simulink model "Benchmark2021ControllerNew"  (R2018a)
settings: Solver=ode1  StartTime=0  StopTime=t_end  FixedStep=simTs  RelTol=1e-3
values from neighbouring files (symbols this model uses):
  Horizon_Lowlayer = T_PreDomn-T_Apply    [Initial_Lower.m]
  Initial_headway = Sensor_FOL_dDist(2)    [Initial_main.m]
  Initial_MG1_spd = 0    [Initial_Lower.m]
  Initial_MG2_spd = 0    [Initial_Lower.m]
  Initial_SOC = 50    [Initial_main.m]
  Initial_vhcl_spd = 0    [Initial_main.m]
  N_opt = zeros(1,length(Power_ex))    [Initial_Lower.m]
  N_PMP_Lowlayer = Horizon_Lowlayer/Sampling_Lowlayer    [Initial_Lower.m]
  Power_level = 0:200:62800    [Initial_Lower.m]
  ras2rpm = 60/2/pi    (= 9.54929658551)    [Initial_main.m]
  Route_Destination_Distance = 16002    [Initial_Upper.m]
  rpm2rads = 1/rads2rpm    (= 0.10471975512)    [Initial_Lower.m]    (also in Initial_main.m)
  Sampling_Lowlayer = 0.05    [Initial_Lower.m]
  T_opt = zeros(1,length(Power_ex))    [Initial_Lower.m]
undefined symbols (not defined in the file or in its folder): DiscIntNeverNeededParam, Maxtorque_EngTrq, MG2_MaxMintorque_MaxTrq, MG2_MaxMintorque_Spd, Rc2, Rf1, Rf2, Rm, Rt, UpperLayerVpredict
(part 1 of 11)
settings Model: PauseTimes=100  Creator=1562880  LastModifiedBy=Lenovo
settings DataIOCC: SaveFormat=Structure  SaveOutput=off  SignalLogging=off  DSMLogging=off  SaveTime=off
settings OptimizationCC: BooleanDataType=off  DefaultParameterBehavior=Inlined  LifeSpan=1
settings DebuggingCC: SolverPrmCheckMsg=warning  FcnCallInpInsideContextMsg=warning  StateNameClashWarn=warning  SFUnexpectedBacktrackingDiag=warning  SFNoUnconditionalDefaultTransitionDiag=warning  SFExecutionAtInitializationDiag=none
settings CodeAppCC: StateflowObjectComments=on
settings GRTTargetCC: TargetLangStandard=C89/C90 (ANSI)  GeneratePreprocessorConditionals=Disable all
settings ConfigComp: CovMetricSettings=dw  CovHtmlReporting=on  CovSaveCumulativeToWorkspaceVar=on  CovSaveSingleToWorkspaceVar=on  CovExternalEMLEnable=off

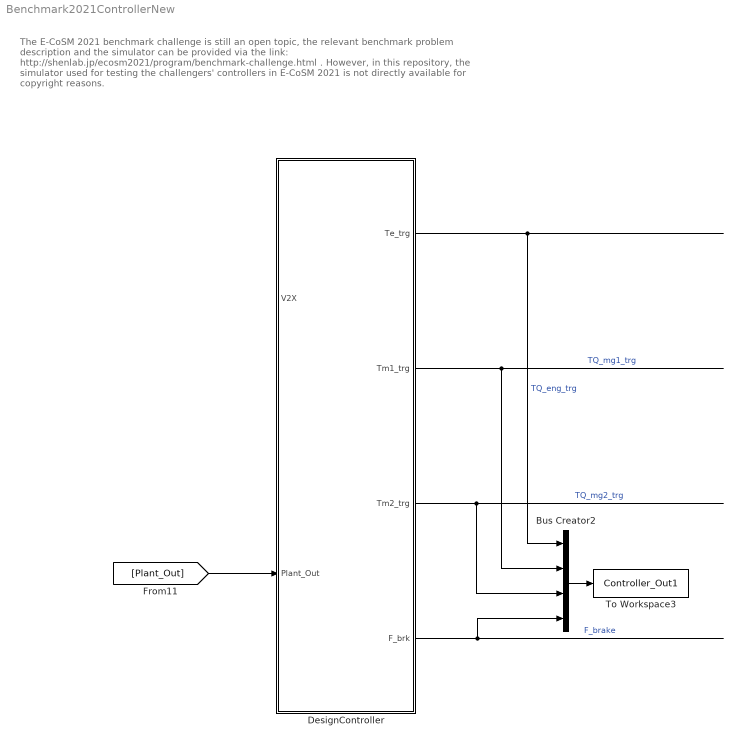
== system Benchmark2021ControllerNew ==
  note: The E-CoSM 2021 benchmark challenge is still an open topic, the relevant benchmark problem description and the simulator can be provided via the link: http://shenlab.jp/ecosm2021/program/benchmark-challenge.html . However, in this repository, the simulator used for testing the challengers' controllers in E-CoSM 2021 is not directly available for copyright reasons.
  Bus Creator2 : BusCreator  Inputs=4
  DesignController : Subsystem
  To Workspace3 : ToWorkspace  VariableName=Controller_Out1  SaveFormat=Timeseries  SampleTime=-1
  wires:
  [Plant_Out] -> DesignController/2(Plant_Out)
  DesignController/3(Tm2_trg) -> Bus Creator2/3  "TQ_mg2_trg"
  Bus Creator2/1 -> To Workspace3/1
  DesignController/1(Te_trg) -> Bus Creator2/1  "TQ_eng_trg"
  DesignController/4(F_brk) -> Bus Creator2/4  "F_brake"
  DesignController/2(Tm1_trg) -> Bus Creator2/2  "TQ_mg1_trg"

== system Benchmark2021ControllerNew/DesignController ==
  V2X : Inport
  Plant_Out : Inport  Port=2
  Benchmark-Controller : Subsystem
      mask Display: disp('JLU\nController')
  Te_trg : Outport
  Tm1_trg : Outport  Port=2
  Tm2_trg : Outport  Port=3
  F_brk : Outport  Port=4
  wires:
  V2X/1 -> Benchmark-Controller/1(V2X)  "Vel_trg"
  Benchmark-Controller/1(Te_trg) -> Te_trg/1
  Benchmark-Controller/2(Tm1_trg) -> Tm1_trg/1
  Benchmark-Controller/3(Tm2_trg) -> Tm2_trg/1
  Benchmark-Controller/4(F_brk) -> F_brk/1
  Plant_Out/1 -> Benchmark-Controller/2(Plant_Out)  "from E-CoSM plant-output"

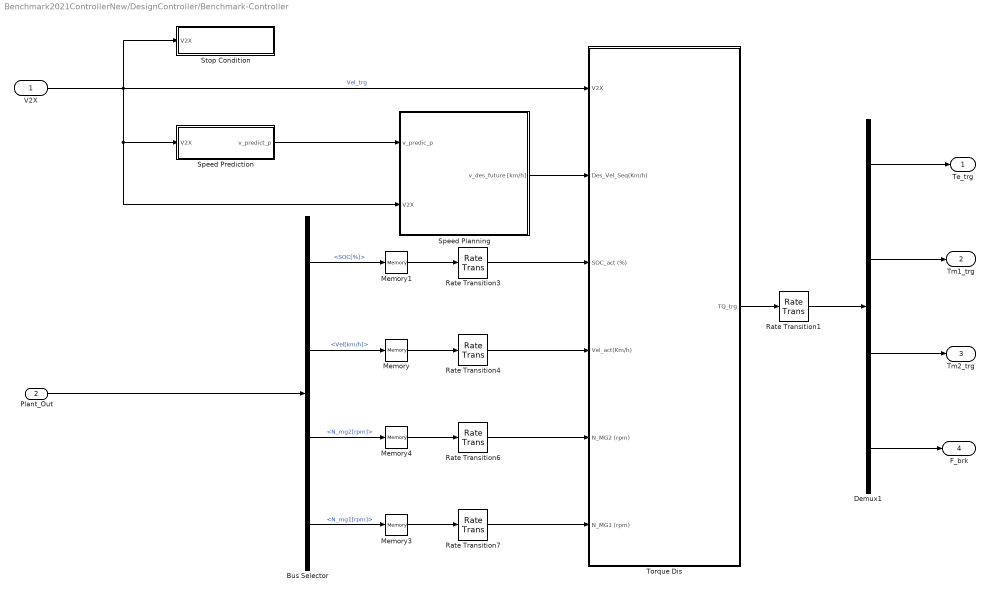
== system Benchmark2021ControllerNew/DesignController/Benchmark-Controller ==
  V2X : Inport
  Plant_Out : Inport  Port=2
  Bus Selector : BusSelector  OutputSignals=SOC[%],Vel[km/h],N_mg2[rpm],N_mg1[rpm]
  Demux1 : Demux
  Memory : Memory  InitialCondition=Initial_vhcl_spd
  Memory1 : Memory  InitialCondition=Initial_SOC
  Memory3 : Memory  InitialCondition=Initial_MG1_spd
  Memory4 : Memory  InitialCondition=Initial_MG2_spd
  Rate Transition1 : RateTransition  OutPortSampleTime=0.01
  Rate Transition3 : RateTransition  InitialCondition=50  OutPortSampleTime=0.05
  Rate Transition4 : RateTransition  OutPortSampleTime=0.05
  Rate Transition6 : RateTransition  OutPortSampleTime=0.05
  Rate Transition7 : RateTransition  OutPortSampleTime=0.05
  Speed Planning : Subsystem
  Speed Prediction : Subsystem  SystemSampleTime=0.05
  Stop Condition : Subsystem
  Torque Dis : Subsystem  SystemSampleTime=0.05
  Te_trg : Outport
  Tm1_trg : Outport  Port=2
  Tm2_trg : Outport  Port=3
  F_brk : Outport  Port=4
  wires:
  Speed Prediction/1(v_predict_p) -> Speed Planning/1(v_predic_p)
  V2X/1 -> Speed Planning/2(V2X), Speed Prediction/1(V2X), Stop Condition/1(V2X), Torque Dis/1(V2X)  "Vel_trg"
  Demux1/1 -> Te_trg/1
  Speed Planning/1(v_des_future [km/h]) -> Torque Dis/2(Des_Vel_Seq(Km/h))
  Torque Dis/1(TQ_trg) -> Rate Transition1/1
  Memory1/1 -> Rate Transition3/1
  Demux1/3 -> Tm2_trg/1
  Memory4/1 -> Rate Transition6/1
  Memory3/1 -> Rate Transition7/1
  Memory/1 -> Rate Transition4/1
  Demux1/4 -> F_brk/1
  Demux1/2 -> Tm1_trg/1
  Plant_Out/1 -> Bus Selector/1
  Bus Selector/1 -> Memory1/1  "<SOC[%]>"
  Bus Selector/2 -> Memory/1  "<Vel[km/h]>"
  Bus Selector/3 -> Memory4/1  "<N_mg2[rpm]>"
  Bus Selector/4 -> Memory3/1  "<N_mg1[rpm]>"
  Rate Transition3/1 -> Torque Dis/3(SOC_act (%))
  Rate Transition4/1 -> Torque Dis/4(Vel_act(Km/h))
  Rate Transition6/1 -> Torque Dis/5(N_MG2 (rpm))
  Rate Transition7/1 -> Torque Dis/6(N_MG1 (rpm))
  Rate Transition1/1 -> Demux1/1

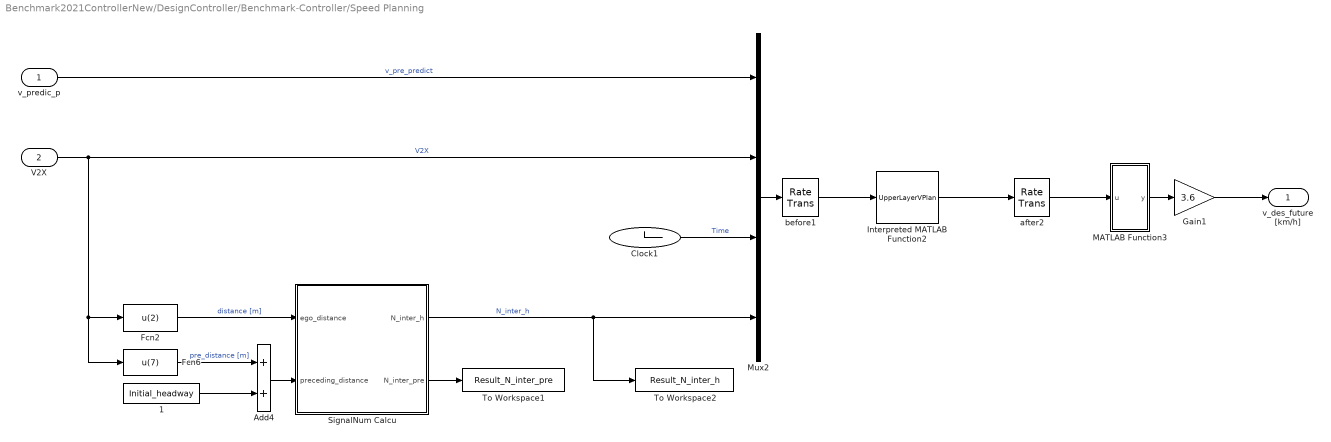
== system Benchmark2021ControllerNew/DesignController/Benchmark-Controller/Speed Planning ==
  v_predic_p : Inport
  V2X : Inport  Port=2
  " 1" : Constant  Value=Initial_headway
  Add4 : Sum
  Clock1 : Clock
  Fcn2 : Fcn  Expr=u(2)
  Fcn6 : Fcn  Expr=u(7)
  Gain1 : Gain  Gain=3.6
  Interpreted MATLAB Function2 : MATLABFcn  MATLABFcn=UpperLayerVPlan  Output1D=off
  MATLAB Function3 : MATLAB Function  TreatAsAtomicUnit=on
  Mux2 : Mux
  SignalNum Calcu : MATLAB Function  TreatAsAtomicUnit=on
  To Workspace1 : ToWorkspace  VariableName=Result_N_inter_pre  SampleTime=-1
      settings: Save2DSignal=2-D array (concatenate along first dimension)
  To Workspace2 : ToWorkspace  VariableName=Result_N_inter_h  SampleTime=-1
      settings: Save2DSignal=2-D array (concatenate along first dimension)
  after2 : RateTransition  OutPortSampleTime=simTs
  before1 : RateTransition  OutPortSampleTime=Ts_upper
  v_des_future [km/h] : Outport
  wires:
  Interpreted MATLAB Function2/1 -> after2/1
  MATLAB Function3/1(y) -> Gain1/1
  after2/1 -> MATLAB Function3/1(u)
  before1/1 -> Interpreted MATLAB Function2/1
  v_predic_p/1 -> Mux2/1  "v_pre_predict"
  Mux2/1 -> before1/1
  Clock1/1 -> Mux2/3  "Time"
  SignalNum Calcu/1(N_inter_h) -> Mux2/4, To Workspace2/1  "N_inter_h"
  Gain1/1 -> v_des_future [km/h]/1
  " 1"/1 -> Add4/2
  Add4/1 -> SignalNum Calcu/2(preceding_distance)
  V2X/1 -> Mux2/2, Fcn6/1, Fcn2/1  "V2X"
  Fcn6/1 -> Add4/1  "pre_distance [m]"
  Fcn2/1 -> SignalNum Calcu/1(ego_distance)  "distance [m]"
  SignalNum Calcu/2(N_inter_pre) -> To Workspace1/1

== system Benchmark2021ControllerNew/DesignController/Benchmark-Controller/Speed Prediction ==
  V2X : Inport
  Clock1 : Clock
  Delay : Subsystem
  Interpreted MATLAB Function : MATLABFcn  MATLABFcn=UpperLayerVpredict(u(1:20),u(21))
  MATLAB Function1 : MATLAB Function  TreatAsAtomicUnit=on
  Mux : Mux  Inputs=2
  after1 : RateTransition  OutPortSampleTime=simTs
  before3 : RateTransition  OutPortSampleTime=Ts_predict
  before4 : RateTransition  OutPortSampleTime=Ts_predict
  v_pre [m/s] : Fcn  Expr=u(6)
  v_predict_p : Outport
  wires:
  Interpreted MATLAB Function/1 -> after1/1
  before3/1 -> Mux/2
  before4/1 -> Delay/1(In1)
  Clock1/1 -> before3/1
  Mux/1 -> Interpreted MATLAB Function/1
  Delay/1(Out1) -> Mux/1
  V2X/1 -> v_pre [m/s]/1
  v_pre [m/s]/1 -> before4/1
  after1/1 -> MATLAB Function1/1(u)
  MATLAB Function1/1(y) -> v_predict_p/1

== system Benchmark2021ControllerNew/DesignController/Benchmark-Controller/Stop Condition ==
  V2X : Inport
  Constant : Constant  Value=Route_Destination_Distance
  Relational Operator : RelationalOperator  OutDataTypeStr=boolean  RndMeth=Simplest
  Stop Simulation : Stop
  s_h [m] : Fcn  Expr=u(2)
  wires:
  V2X/1 -> s_h [m]/1
  Constant/1 -> Relational Operator/2
  s_h [m]/1 -> Relational Operator/1
  Relational Operator/1 -> Stop Simulation/1

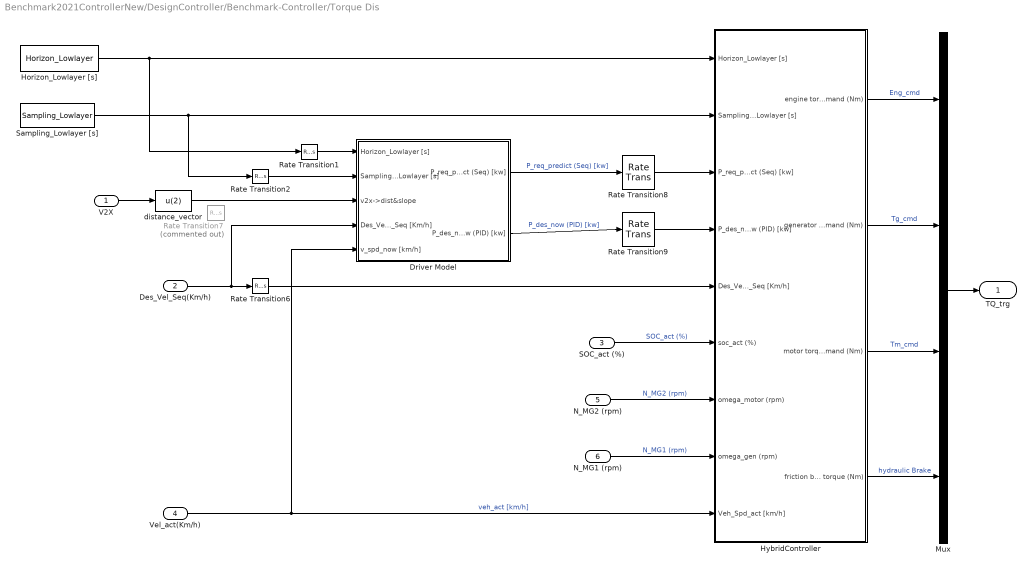
== system Benchmark2021ControllerNew/DesignController/Benchmark-Controller/Torque Dis ==
  V2X : Inport
  Des_Vel_Seq(Km/h) : Inport  Port=2
  SOC_act (%) : Inport  Port=3
  Vel_act(Km/h) : Inport  Port=4
  N_MG2 (rpm) : Inport  Port=5
  N_MG1 (rpm) : Inport  Port=6
  Driver Model : Subsystem
  Horizon_Lowlayer [s] : Constant  Value=Horizon_Lowlayer
  HybridController : Subsystem  SystemSampleTime=0.05
      mask Display: disp('Torque Distribution\nController')
  Mux : Mux
  Rate Transition1 : RateTransition  OutPortSampleTime=0.01
  Rate Transition2 : RateTransition  OutPortSampleTime=0.01
  Rate Transition6 : RateTransition  OutPortSampleTime=0.05
  Rate Transition7 : RateTransition  Commented=on  OutPortSampleTime=0.05
  Rate Transition8 : RateTransition  OutPortSampleTime=0.05
  Rate Transition9 : RateTransition  OutPortSampleTime=0.05
  Sampling_Lowlayer [s] : Constant  Value=Sampling_Lowlayer
  distance_vector : Fcn  Expr=u(2)
  TQ_trg : Outport
  wires:
  N_MG1 (rpm)/1 -> HybridController/8(omega_gen (rpm))  "N_MG1 (rpm)"
  N_MG2 (rpm)/1 -> HybridController/7(omega_motor (rpm))  "N_MG2 (rpm)"
  SOC_act (%)/1 -> HybridController/6(soc_act (%))  "SOC_act (%)"
  HybridController/4(friction brake torque (Nm)) -> Mux/4  "hydraulic Brake"
  Driver Model/2(P_des_now (PID) [kw]) -> Rate Transition9/1  "P_des_now (PID) [kw]"
  Mux/1 -> TQ_trg/1
  HybridController/1(engine torque command (Nm)) -> Mux/1  "Eng_cmd"
  HybridController/2(generator torque command (Nm)) -> Mux/2  "Tg_cmd"
  HybridController/3(motor torque command (Nm)) -> Mux/3  "Tm_cmd"
  Driver Model/1(P_req_predict (Seq) [kw]) -> Rate Transition8/1  "P_req_predict (Seq) [kw]"
  V2X/1 -> distance_vector/1
  Vel_act(Km/h)/1 -> Driver Model/5(v_spd_now [km/h]), HybridController/9(Veh_Spd_act [km/h])  "veh_act [km/h]"
  Des_Vel_Seq(Km/h)/1 -> Driver Model/4(Des_VehSpd_Seq [Km/h]), Rate Transition6/1
  Horizon_Lowlayer [s]/1 -> HybridController/1(Horizon_Lowlayer [s]), Rate Transition1/1
  Sampling_Lowlayer [s]/1 -> Rate Transition2/1, HybridController/2(Sampling_Lowlayer [s])
  distance_vector/1 -> Driver Model/3(v2x->dist&slope)
  Rate Transition6/1 -> HybridController/5(Des_VehSpd_Seq [Km/h])
  Rate Transition9/1 -> HybridController/4(P_des_now (PID) [kw])
  Rate Transition8/1 -> HybridController/3(P_req_predict (Seq) [kw])
  Rate Transition1/1 -> Driver Model/1(Horizon_Lowlayer [s])
  Rate Transition2/1 -> Driver Model/2(Sampling_Lowlayer [s])

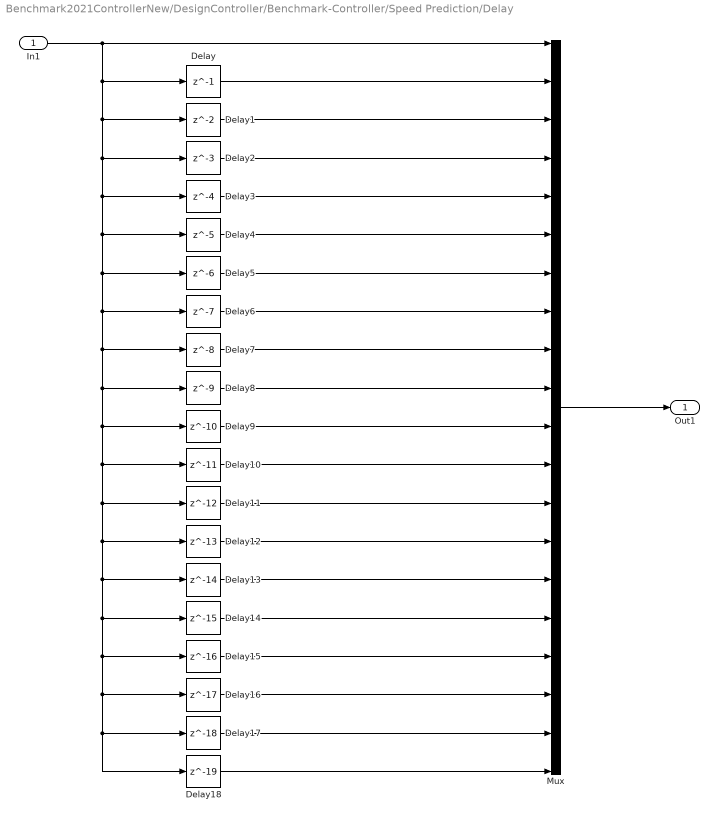
== system Benchmark2021ControllerNew/DesignController/Benchmark-Controller/Speed Prediction/Delay ==
  In1 : Inport
  Delay : Delay  DelayLength=1
  Delay1 : Delay
  Delay10 : Delay  DelayLength=11
  Delay11 : Delay  DelayLength=12
  Delay12 : Delay  DelayLength=13
  Delay13 : Delay  DelayLength=14
  Delay14 : Delay  DelayLength=15
  Delay15 : Delay  DelayLength=16
  Delay16 : Delay  DelayLength=17
  Delay17 : Delay  DelayLength=18
  Delay18 : Delay  DelayLength=19
  Delay2 : Delay  DelayLength=3
  Delay3 : Delay  DelayLength=4
  Delay4 : Delay  DelayLength=5
  Delay5 : Delay  DelayLength=6
  Delay6 : Delay  DelayLength=7
  Delay7 : Delay  DelayLength=8
  Delay8 : Delay  DelayLength=9
  Delay9 : Delay  DelayLength=10
  Mux : Mux  Inputs=20
  Out1 : Outport
  wires:
  Delay8/1 -> Mux/10
  Delay10/1 -> Mux/12
  In1/1 -> Delay14/1, Delay17/1, Delay18/1, Delay16/1, Delay15/1, Delay13/1, Delay12/1, Delay11/1, Delay10/1, Delay9/1, Delay8/1, Delay7/1, Delay6/1, Delay5/1, Delay4/1, Delay3/1, Delay2/1, Delay1/1, Delay/1, Mux/1
  Delay11/1 -> Mux/13
  Delay2/1 -> Mux/4
  Delay7/1 -> Mux/9
  Delay15/1 -> Mux/17
  Delay9/1 -> Mux/11
  Delay12/1 -> Mux/14
  Delay13/1 -> Mux/15
  Delay14/1 -> Mux/16
  Delay4/1 -> Mux/6
  Delay16/1 -> Mux/18
  Delay6/1 -> Mux/8
  Delay5/1 -> Mux/7
  Delay17/1 -> Mux/19
  Delay18/1 -> Mux/20
  Delay/1 -> Mux/2
  Delay3/1 -> Mux/5
  Delay1/1 -> Mux/3
  Mux/1 -> Out1/1

== system Benchmark2021ControllerNew/DesignController/Benchmark-Controller/Torque Dis/Driver Model ==
  Horizon_Lowlayer [s] : Inport  SampleTime=0.05
  Sampling_Lowlayer [s] : Inport  Port=2  SampleTime=0.05
  v2x->dist&slope : Inport  Port=3
  Des_VehSpd_Seq [Km/h] : Inport  Port=4
  v_spd_now [km/h] : Inport  Port=5
  B4 - PID : Subsystem
  Fcn : Fcn  Expr=u(1)
  Power_cal : Subsystem
  To Workspace21 : ToWorkspace  VariableName=Data_Pdes_now  SampleTime=0.05
  Unit Delay : UnitDelay  SampleTime=0.05
  P_req_predict (Seq) [kw] : Outport
  P_des_now (PID) [kw] : Outport  Port=2
  wires:
  Power_cal/2(Power_des_now [kw]) -> To Workspace21/1, P_des_now (PID) [kw]/1  "P-des_now ( with PID) [kw]"
  Sampling_Lowlayer [s]/1 -> Power_cal/2(Sampling_Lowlayer [s])
  Horizon_Lowlayer [s]/1 -> Power_cal/1(Horizon_Lowlayer [s])
  Unit Delay/1 -> Power_cal/4(Dist_init [m])
  v2x->dist&slope/1 -> Unit Delay/1
  Power_cal/1(P_req_predict (Seq) [kw]) -> P_req_predict (Seq) [kw]/1  "P_req-MPC [kw]"
  Fcn/1 -> B4 - PID/1(v_des_now [km/h])  "Des_VehSpd [km/h]"
  v_spd_now [km/h]/1 -> B4 - PID/2(v_real_now [km/h])  "v_spd_now [km/h]"
  B4 - PID/1(delta Power [kw]) -> Power_cal/5(P_only_PID [kw])  "TQ-OnlyPID [kw]"
  Des_VehSpd_Seq [Km/h]/1 -> Power_cal/3(Seq_v_des_req [km/h]), Fcn/1  "Seq_v_des_req [km/h]"

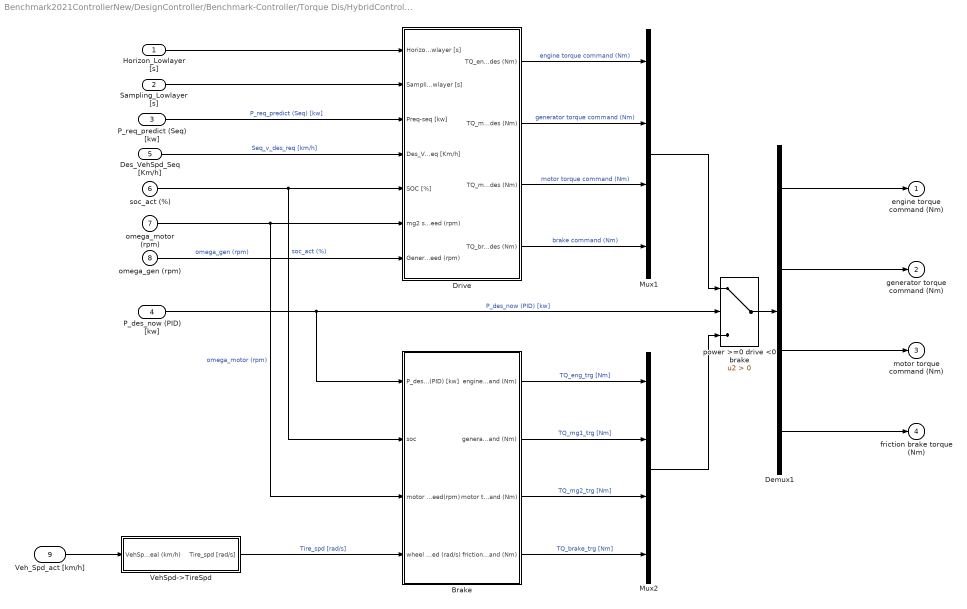
== system Benchmark2021ControllerNew/DesignController/Benchmark-Controller/Torque Dis/HybridController ==
  Horizon_Lowlayer [s] : Inport  SampleTime=0.05
  Sampling_Lowlayer [s] : Inport  Port=2  SampleTime=0.05
  P_req_predict (Seq) [kw] : Inport  Port=3
  P_des_now (PID) [kw] : Inport  Port=4
  Des_VehSpd_Seq [Km/h] : Inport  Port=5
  soc_act (%) : Inport  Port=6
  omega_motor (rpm) : Inport  Port=7
  omega_gen (rpm) : Inport  Port=8
  Veh_Spd_act [km/h] : Inport  Port=9
  Brake : Subsystem  AncestorBlock=|
      | lib_controls/<vc> prius/Coordinated
      |  Controller/max engine
      | efficiency point
      mask Display: disp('Braking\nControl')
  Demux1 : Demux
  Drive : Subsystem  AncestorBlock=|
      | lib_controls/<vc> prius/Coordinated
      |  Controller/max engine
      | efficiency point
      mask Display: disp('Driving\nControl')
  Mux1 : Mux
  Mux2 : Mux
  VehSpd->TireSpd : Subsystem
  power >=0 drive <0 brake : Switch  Criteria=u2 > Threshold  SaturateOnIntegerOverflow=on
  engine torque command (Nm) : Outport
  generator torque command (Nm) : Outport  Port=2
  motor torque command (Nm) : Outport  Port=3
  friction brake torque (Nm) : Outport  Port=4
  wires:
  Drive/3(TQ_mg2_des (Nm)) -> Mux1/3  "motor torque command (Nm)"
  soc_act (%)/1 -> Brake/2(soc), Drive/5(SOC [%])  "soc_act (%)"
  Mux1/1 -> power >=0 drive <0 brake/1
  Drive/1(TQ_eng_des (Nm)) -> Mux1/1  "engine torque command (Nm)"
  P_des_now (PID) [kw]/1 -> Brake/1(P_des_now (PID) [kw]), power >=0 drive <0 brake/2  "P_des_now (PID) [kw]"
  Drive/2(TQ_mg1_des (Nm)) -> Mux1/2  "generator torque command (Nm)"
  Drive/4(TQ_brake_des (Nm)) -> Mux1/4  "brake command (Nm)"
  Demux1/1 -> engine torque command (Nm)/1
  omega_motor (rpm)/1 -> Brake/3(motor speed(rpm)), Drive/6(mg2 speed (rpm))  "omega_motor (rpm)"
  omega_gen (rpm)/1 -> Drive/7(Generator speed (rpm))  "omega_gen (rpm)"
  Demux1/2 -> generator torque command (Nm)/1
  Demux1/3 -> motor torque command (Nm)/1
  Demux1/4 -> friction brake torque (Nm)/1
  power >=0 drive <0 brake/1 -> Demux1/1
  VehSpd->TireSpd/1(Tire_spd [rad/s]) -> Brake/4(wheel speed (rad/s))  "Tire_spd [rad/s]"
  P_req_predict (Seq) [kw]/1 -> Drive/3(Preq-seq [kw])  "P_req_predict (Seq) [kw]"
  Veh_Spd_act [km/h]/1 -> VehSpd->TireSpd/1(VehSpd_real (km/h))
  Brake/1(engine torque command (Nm)) -> Mux2/1  "TQ_eng_trg [Nm]"
  Brake/2(generator torque command (Nm)) -> Mux2/2  "TQ_mg1_trg [Nm]"
  Brake/3(motor torque command (Nm)) -> Mux2/3  "TQ_mg2_trg [Nm]"
  Brake/4(friction brake torque command (Nm)) -> Mux2/4  "TQ_brake_trg [Nm]"
  Mux2/1 -> power >=0 drive <0 brake/3
  Des_VehSpd_Seq [Km/h]/1 -> Drive/4(Des_VehSpd_Seq [Km/h])  "Seq_v_des_req [km/h]"
  Horizon_Lowlayer [s]/1 -> Drive/1(Horizon_Lowlayer [s])
  Sampling_Lowlayer [s]/1 -> Drive/2(Sampling_Lowlayer [s])

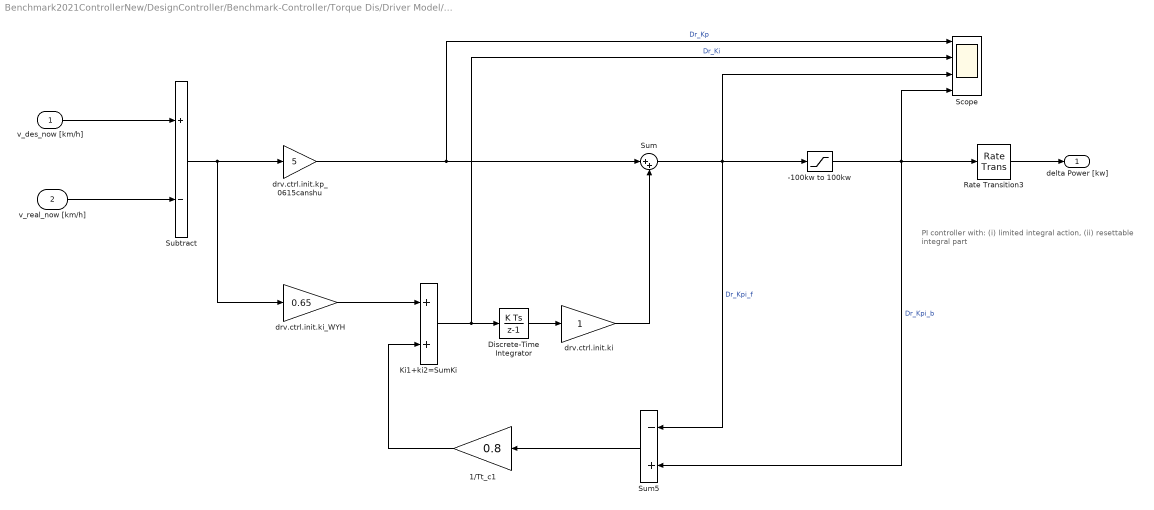
== system Benchmark2021ControllerNew/DesignController/Benchmark-Controller/Torque Dis/Driver Model/B4 - PID ==
  note: PI controller with:
      | (i) limited integral action,
      | (ii) resettable integral part
  v_des_now [km/h] : Inport
  v_real_now [km/h] : Inport  Port=2
  "-100kw to 100kw " : Saturate  UpperLimit=20  LowerLimit=-100
  1/Tt_c1 : Gain  Gain=0.8  SaturateOnIntegerOverflow=on  OutDataTypeStr=Inherit: Same as input  ParamDataTypeStr=Inherit: Same as input
  Discrete-Time Integrator : DiscreteIntegrator  SampleTime=0.05  ICPrevOutput=DiscIntNeverNeededParam  ICPrevScaledInput=DiscIntNeverNeededParam
  Ki1+ki2=SumKi : Sum  SaturateOnIntegerOverflow=on  InputSameDT=on  OutDataTypeStr=Inherit: Same as first input
  Rate Transition3 : RateTransition  OutPortSampleTime=0.05
  Scope : Scope  NumInputPorts=4
  Subtract : Sum  Inputs=+-
  Sum : Sum  Inputs=|++  SaturateOnIntegerOverflow=on  InputSameDT=on  OutDataTypeStr=Inherit: Same as first input
  Sum5 : Sum  Inputs=-+  SaturateOnIntegerOverflow=on  InputSameDT=on  OutDataTypeStr=Inherit: Same as first input
  drv.ctrl.init.ki : Gain  SaturateOnIntegerOverflow=on  OutDataTypeStr=Inherit: Same as input  ParamDataTypeStr=Inherit: Same as input
  drv.ctrl.init.ki_WYH : Gain  Gain=0.65  SaturateOnIntegerOverflow=on  OutDataTypeStr=Inherit: Same as input  ParamDataTypeStr=Inherit: Same as input
  drv.ctrl.init.kp_0615canshu : Gain  Gain=5  SaturateOnIntegerOverflow=on  OutDataTypeStr=Inherit: Same as input  ParamDataTypeStr=Inherit: Same as input
  delta Power [kw] : Outport
  wires:
  drv.ctrl.init.kp_0615canshu/1 -> Sum/1, Scope/1  "Dr_Kp"
  drv.ctrl.init.ki_WYH/1 -> Ki1+ki2=SumKi/1
  1/Tt_c1/1 -> Ki1+ki2=SumKi/2
  Sum/1 -> "-100kw to 100kw "/1, Scope/3, Sum5/1  "Dr_Kpi_f"
  Ki1+ki2=SumKi/1 -> Discrete-Time Integrator/1, Scope/2  "Dr_Ki"
  Sum5/1 -> 1/Tt_c1/1
  Subtract/1 -> drv.ctrl.init.ki_WYH/1, drv.ctrl.init.kp_0615canshu/1
  "-100kw to 100kw "/1 -> Rate Transition3/1, Scope/4, Sum5/2  "Dr_Kpi_b"
  drv.ctrl.init.ki/1 -> Sum/2
  Discrete-Time Integrator/1 -> drv.ctrl.init.ki/1
  v_des_now [km/h]/1 -> Subtract/1
  v_real_now [km/h]/1 -> Subtract/2
  Rate Transition3/1 -> delta Power [kw]/1

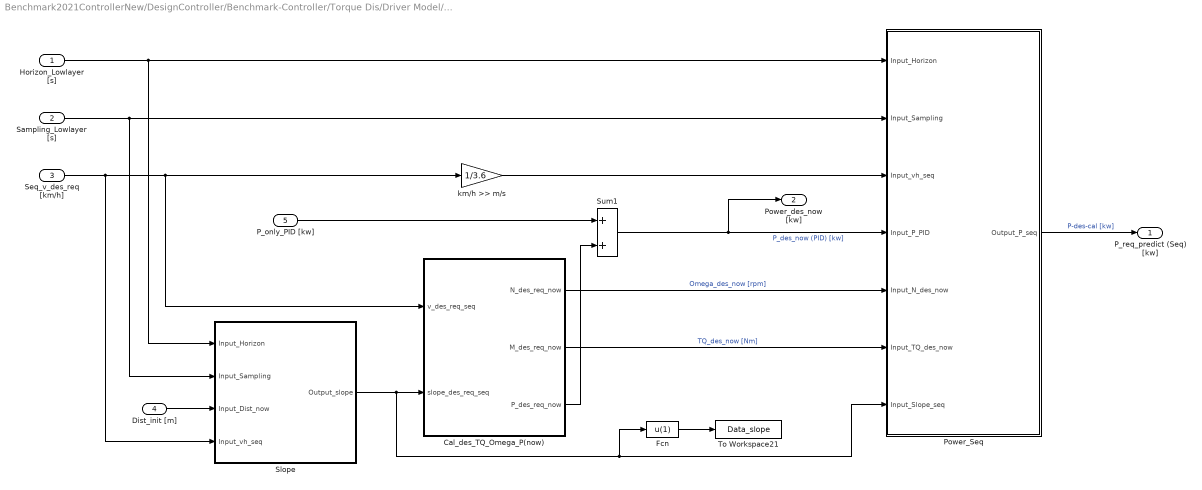
== system Benchmark2021ControllerNew/DesignController/Benchmark-Controller/Torque Dis/Driver Model/Power_cal ==
  Horizon_Lowlayer [s] : Inport  SampleTime=0.05
  Sampling_Lowlayer [s] : Inport  Port=2  SampleTime=0.05
  Seq_v_des_req [km/h] : Inport  Port=3  SampleTime=0.05
  Dist_init [m] : Inport  Port=4  SampleTime=0.05
  P_only_PID [kw] : Inport  Port=5  SampleTime=0.05
  Cal_des_TQ_Omega_P(now) : MATLAB Function  TreatAsAtomicUnit=on
  Fcn : Fcn  Expr=u(1)
  Power_Seq : MATLAB Function  TreatAsAtomicUnit=on
  Slope : MATLAB Function  TreatAsAtomicUnit=on
  Sum1 : Sum  SaturateOnIntegerOverflow=on  InputSameDT=on  OutDataTypeStr=Inherit: Same as first input
  To Workspace21 : ToWorkspace  VariableName=Data_slope  SampleTime=0.05
  km/h >> m/s : Gain  Gain=1/3.6
  P_req_predict (Seq) [kw] : Outport
  Power_des_now [kw] : Outport  Port=2
  wires:
  Cal_des_TQ_Omega_P(now)/3(P_des_req_now) -> Sum1/2
  Dist_init [m]/1 -> Slope/3(Input_Dist_now)
  P_only_PID [kw]/1 -> Sum1/1
  Power_Seq/1(Output_P_seq) -> P_req_predict (Seq) [kw]/1  "P-des-cal [kw]"
  Sum1/1 -> Power_Seq/4(Input_P_PID), Power_des_now [kw]/1  "P_des_now (PID) [kw]"
  km/h >> m/s/1 -> Power_Seq/3(Input_vh_seq)
  Horizon_Lowlayer [s]/1 -> Power_Seq/1(Input_Horizon), Slope/1(Input_Horizon)
  Seq_v_des_req [km/h]/1 -> Slope/4(Input_vh_seq), km/h >> m/s/1, Cal_des_TQ_Omega_P(now)/1(v_des_req_seq)
  Sampling_Lowlayer [s]/1 -> Slope/2(Input_Sampling), Power_Seq/2(Input_Sampling)
  Cal_des_TQ_Omega_P(now)/2(M_des_req_now) -> Power_Seq/6(Input_TQ_des_now)  "TQ_des_now [Nm]"
  Cal_des_TQ_Omega_P(now)/1(N_des_req_now) -> Power_Seq/5(Input_N_des_now)  "Omega_des_now [rpm]"
  Slope/1(Output_slope) -> Fcn/1, Power_Seq/7(Input_Slope_seq), Cal_des_TQ_Omega_P(now)/2(slope_des_req_seq)
  Fcn/1 -> To Workspace21/1

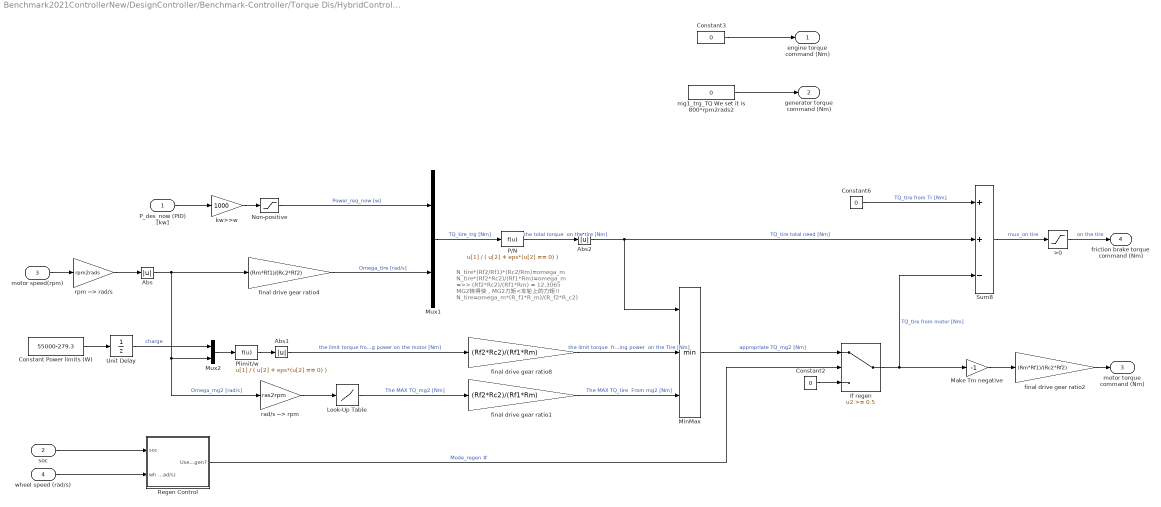
== system Benchmark2021ControllerNew/DesignController/Benchmark-Controller/Torque Dis/HybridController/Brake ==
  note: N_tire*(Rf2/Rf1)*(Rc2/Rm)=omega_m
      | N_tire*(Rf2*Rc2)/(Rf1*Rm)=omega_m
      |
      | =>> (Rf2*Rc2)/(Rf1*Rm) = 12.3065
      | MG2转得快，MG2力矩<车轮上的力矩!!
      | N_tire=omega_m*(R_f1*R_m)/(R_f2*R_c2)
  P_des_now (PID) [kw] : Inport
  soc : Inport  Port=2
  motor speed(rpm) : Inport  Port=3
  wheel speed (rad/s) : Inport  Port=4
  " rad/s --> rpm" : Gain  Gain=ras2rpm  SaturateOnIntegerOverflow=on  OutDataTypeStr=Inherit: Same as input  ParamDataTypeStr=Inherit: Same as input
  >0 : Saturate  UpperLimit=20000  LowerLimit=0
  Abs : Abs  SaturateOnIntegerOverflow=on
  Abs1 : Abs  SaturateOnIntegerOverflow=on
  Abs2 : Abs  SaturateOnIntegerOverflow=on
  Constant Power limits (W) : Constant  Value=55000-279.3
  Constant2 : Constant  Value=0
  Constant3 : Constant  Value=0
  Constant6 : Constant  Value=0
  If regen : Switch  Threshold=0.5  SaturateOnIntegerOverflow=on  InputSameDT=on
  Look-Up Table : Lookup  InputValues=MG2_MaxMintorque_Spd  Table=MG2_MaxMintorque_MaxTrq  SaturateOnIntegerOverflow=on
  Make Tm negative : Gain  Gain=-1  SaturateOnIntegerOverflow=on  OutDataTypeStr=Inherit: Same as input  ParamDataTypeStr=Inherit: Same as input
  MinMax : MinMax  Inputs=3  SaturateOnIntegerOverflow=on  InputSameDT=on
  Mux1 : Mux  Inputs=2
  Mux2 : Mux  Inputs=2
  Non-positive : Saturate  UpperLimit=0  LowerLimit=-inf
  P/N : Fcn  Expr=u[1] / ( u[2] + eps*(u[2] == 0) )
  Plimit/w : Fcn  Expr=u[1] / ( u[2] + eps*(u[2] == 0) )
  Regen Control : Subsystem
      mask Display: disp('Regen\nControl')
  Sum8 : Sum  Inputs=++-  SaturateOnIntegerOverflow=on  InputSameDT=on  OutDataTypeStr=Inherit: Same as first input
  Unit Delay : UnitDelay  SampleTime=0.05
  final drive gear ratio1 : Gain  Gain=(Rf2*Rc2)/(Rf1*Rm)  SaturateOnIntegerOverflow=on  OutDataTypeStr=Inherit: Same as input  ParamDataTypeStr=Inherit: Same as input
  final drive gear ratio2 : Gain  Gain=(Rm*Rf1)/(Rc2*Rf2)  SaturateOnIntegerOverflow=on  OutDataTypeStr=Inherit: Same as input  ParamDataTypeStr=Inherit: Same as input
  final drive gear ratio4 : Gain  Gain=(Rm*Rf1)/(Rc2*Rf2)  SaturateOnIntegerOverflow=on  OutDataTypeStr=Inherit: Same as input  ParamDataTypeStr=Inherit: Same as input
  final drive gear ratio8 : Gain  Gain=(Rf2*Rc2)/(Rf1*Rm)  SaturateOnIntegerOverflow=on  OutDataTypeStr=Inherit: Same as input  ParamDataTypeStr=Inherit: Same as input
  kw>>w : Gain  Gain=1000  SaturateOnIntegerOverflow=on  OutDataTypeStr=Inherit: Same as input  ParamDataTypeStr=Inherit: Same as input
  mg1_trg_TQ We set it is 800*rpm2rads2 : Constant  Value=0
  rpm --> rad/s : Gain  Gain=rpm2rads  SaturateOnIntegerOverflow=on  OutDataTypeStr=Inherit: Same as input  ParamDataTypeStr=Inherit: Same as input
  engine torque command (Nm) : Outport
  generator torque command (Nm) : Outport  Port=2
  motor torque command (Nm) : Outport  Port=3
  friction brake torque command (Nm) : Outport  Port=4
  wires:
  Mux1/1 -> P/N/1  "TQ_tire_trg [Nm]"
  Non-positive/1 -> Mux1/1  "Power_req_now [w]"
  Constant2/1 -> If regen/3
  MinMax/1 -> If regen/1  "appropriate TQ_mg2 [Nm]"
  Unit Delay/1 -> Mux2/1  "charge"
  motor speed(rpm)/1 -> rpm --> rad/s/1
  Abs/1 -> " rad/s --> rpm"/1, Mux2/2, final drive gear ratio4/1  "Omega_mg2 [rad/s]"
  Sum8/1 -> >0/1  "mux_on tire"
  final drive gear ratio1/1 -> MinMax/3  "The MAX TQ_tire  From mg2 [Nm]"
  wheel speed (rad/s)/1 -> Regen Control/2(wh spd (rad/s))
  Plimit/w/1 -> Abs1/1
  P_des_now (PID) [kw]/1 -> kw>>w/1
  soc/1 -> Regen Control/1(soc)
  >0/1 -> friction brake torque command (Nm)/1  "on the tire"
  final drive gear ratio2/1 -> motor torque command (Nm)/1
  Mux2/1 -> Plimit/w/1
  Regen Control/1("Use regen? ") -> If regen/2  "Mode_regen #"
  Constant Power limits (W)/1 -> Unit Delay/1
  " rad/s --> rpm"/1 -> Look-Up Table/1
  final drive gear ratio8/1 -> MinMax/2  "the limit torque  from the charging power  on the Tire [Nm]"
  Abs2/1 -> Sum8/2, MinMax/1  "TQ_tire total need [Nm]"
  If regen/1 -> Sum8/3, Make Tm negative/1  "TQ_tire from motor [Nm]"
  final drive gear ratio4/1 -> Mux1/2  "Omega_tire [rad/s]"
  Look-Up Table/1 -> final drive gear ratio1/1  "The MAX TQ_mg2 [Nm]"
  Abs1/1 -> final drive gear ratio8/1  "the limit torque from the charging power on the motor [Nm]"
  Make Tm negative/1 -> final drive gear ratio2/1
  Constant3/1 -> engine torque command (Nm)/1
  rpm --> rad/s/1 -> Abs/1
  mg1_trg_TQ We set it is 800*rpm2rads2/1 -> generator torque command (Nm)/1
  Constant6/1 -> Sum8/1  "TQ_tire from Tr [Nm]"
  kw>>w/1 -> Non-positive/1
  P/N/1 -> Abs2/1  "the total torque  on the tire [Nm]"

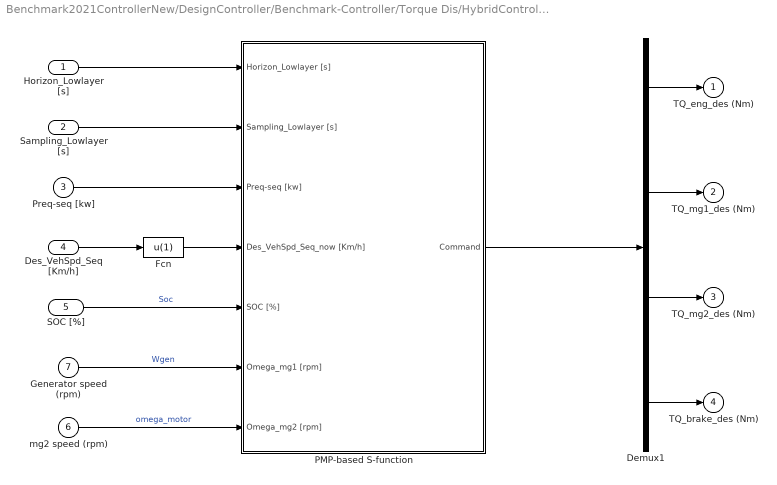
== system Benchmark2021ControllerNew/DesignController/Benchmark-Controller/Torque Dis/HybridController/Drive ==
  Horizon_Lowlayer [s] : Inport  SampleTime=0.05
  Sampling_Lowlayer [s] : Inport  Port=2  SampleTime=0.05
  Preq-seq [kw] : Inport  Port=3
  Des_VehSpd_Seq [Km/h] : Inport  Port=4
  SOC [%] : Inport  Port=5
  mg2 speed (rpm) : Inport  Port=6
  Generator speed (rpm) : Inport  Port=7
  Demux1 : Demux
  Fcn : Fcn  Expr=u(1)
  PMP-based S-function : Subsystem
  TQ_eng_des (Nm) : Outport
  TQ_mg1_des (Nm) : Outport  Port=2
  TQ_mg2_des (Nm) : Outport  Port=3
  TQ_brake_des (Nm) : Outport  Port=4
  wires:
  Preq-seq [kw]/1 -> PMP-based S-function/3(Preq-seq [kw])
  SOC [%]/1 -> PMP-based S-function/5(SOC [%])  "Soc"
  PMP-based S-function/1(Command) -> Demux1/1
  Demux1/1 -> TQ_eng_des (Nm)/1
  Demux1/2 -> TQ_mg1_des (Nm)/1
  Demux1/3 -> TQ_mg2_des (Nm)/1
  Demux1/4 -> TQ_brake_des (Nm)/1
  Des_VehSpd_Seq [Km/h]/1 -> Fcn/1
  Fcn/1 -> PMP-based S-function/4(Des_VehSpd_Seq_now [Km/h])
  Sampling_Lowlayer [s]/1 -> PMP-based S-function/2(Sampling_Lowlayer [s])
  Horizon_Lowlayer [s]/1 -> PMP-based S-function/1(Horizon_Lowlayer [s])
  mg2 speed (rpm)/1 -> PMP-based S-function/7(Omega_mg2 [rpm])  "omega_motor"
  Generator speed (rpm)/1 -> PMP-based S-function/6(Omega_mg1 [rpm])  "Wgen"

== system Benchmark2021ControllerNew/DesignController/Benchmark-Controller/Torque Dis/HybridController/VehSpd->TireSpd ==
  VehSpd_real (km/h) : Inport
  Km/h>>m/s : Gain  Gain=1/3.6
  "because:Rt : mm" : Gain  Gain=1/Rt*1000
  Tire_spd [rad/s] : Outport
  wires:
  VehSpd_real (km/h)/1 -> Km/h>>m/s/1
  Km/h>>m/s/1 -> "because:Rt : mm"/1
  "because:Rt : mm"/1 -> Tire_spd [rad/s]/1

== system Benchmark2021ControllerNew/DesignController/Benchmark-Controller/Torque Dis/HybridController/Brake/Regen Control ==
  note: Rt=317.25mm,
      | Rt*0.4=0.4568km/h
  soc : Inport
  wh spd (rad/s) : Inport  Port=2
  Logical Operator : Logic  Inputs=3
  regen swith on : Constant
  soc condition <=regstop_soc we set it is 70 : Relay  OnSwitchValue=70  OffSwitchValue=70  OnOutputValue=0  OffOutputValue=1
  wheel spd>= 0.4 : Relay  OnSwitchValue=0.4  OffSwitchValue=0.4
  "Use regen? " : Outport
  wires:
  wh spd (rad/s)/1 -> wheel spd>= 0.4/1
  soc/1 -> soc condition <=regstop_soc we set it is 70/1
  Logical Operator/1 -> "Use regen? "/1  "regenmode"
  soc condition <=regstop_soc we set it is 70/1 -> Logical Operator/2
  regen swith on/1 -> Logical Operator/3
  wheel spd>= 0.4/1 -> Logical Operator/1

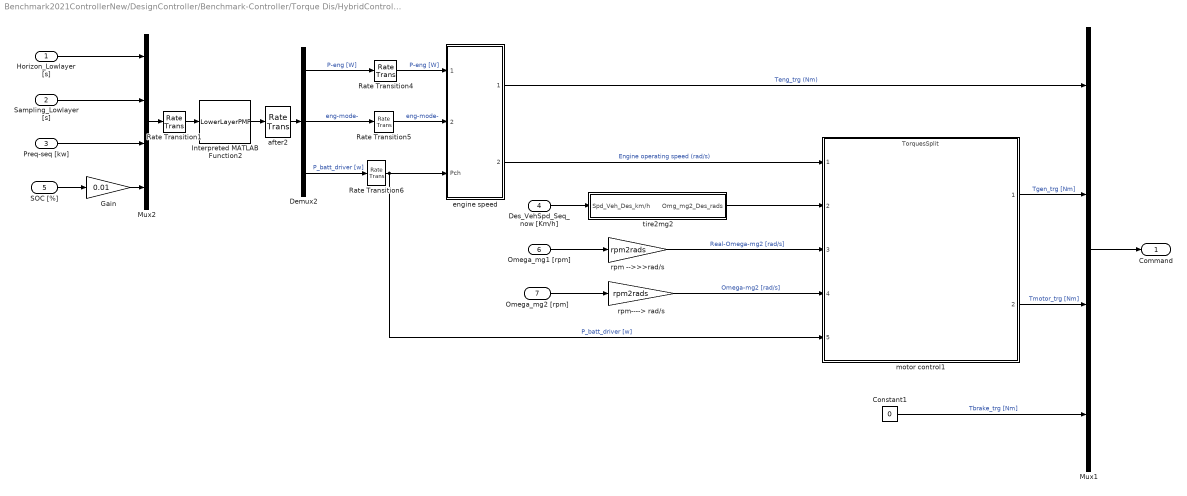
== system Benchmark2021ControllerNew/DesignController/Benchmark-Controller/Torque Dis/HybridController/Drive/PMP-based S-function ==
  Horizon_Lowlayer [s] : Inport  SampleTime=0.05
  Sampling_Lowlayer [s] : Inport  Port=2  SampleTime=0.05
  Preq-seq [kw] : Inport  Port=3
  Des_VehSpd_Seq_now [Km/h] : Inport  Port=4
  SOC [%] : Inport  Port=5
  Omega_mg1 [rpm] : Inport  Port=6
  Omega_mg2 [rpm] : Inport  Port=7
  Constant1 : Constant  Value=0  SampleTime=0.05
  Demux2 : Demux  Outputs=3
  Gain : Gain  Gain=0.01
  Interpreted MATLAB Function2 : MATLABFcn  MATLABFcn=LowerLayerPMP  OutputDimensions=3  Output1D=off
  Mux1 : Mux
  Mux2 : Mux
  Rate Transition{1,4..6} (4 alike) : RateTransition  OutPortSampleTime=0.05
  after2 : RateTransition  OutPortSampleTime=simTs
  engine speed : Subsystem
      mask Display: disp('Engine\nOptimal\nControl')
  motor control1 : ModelReference  ModelNameDialog=TorquesSplit  ModelReferenceVersion=1.659  CopyOfModelProtected=on
  rpm -->>>rad/s : Gain  Gain=rpm2rads  SaturateOnIntegerOverflow=on  OutDataTypeStr=Inherit: Same as input  ParamDataTypeStr=Inherit: Same as input
  rpm----> rad/s : Gain  Gain=rpm2rads  SaturateOnIntegerOverflow=on  OutDataTypeStr=Inherit: Same as input  ParamDataTypeStr=Inherit: Same as input
  tire2mg2 : Subsystem
  Command : Outport
  wires:
  tire2mg2/1(Omg_mg2_Des_rads) -> motor control1/2
  Des_VehSpd_Seq_now [Km/h]/1 -> tire2mg2/1(Spd_Veh_Des_km/h)
  rpm -->>>rad/s/1 -> motor control1/3  "Real-Omega-mg2 [rad/s]"
  rpm----> rad/s/1 -> motor control1/4  "Omega-mg2 [rad/s]"
  engine speed/1(Te (Nm)) -> Mux1/1  "Teng_trg (Nm)"
  engine speed/2(Engine operating speed (rad/s)) -> motor control1/1  "Engine operating speed (rad/s)"
  motor control1/2 -> Mux1/3  "Tmotor_trg [Nm]"
  Constant1/1 -> Mux1/4  "Tbrake_trg [Nm]"
  Mux1/1 -> Command/1
  motor control1/1 -> Mux1/2  "Tgen_trg [Nm]"
  Omega_mg1 [rpm]/1 -> rpm -->>>rad/s/1
  Omega_mg2 [rpm]/1 -> rpm----> rad/s/1
  Preq-seq [kw]/1 -> Mux2/3
  Sampling_Lowlayer [s]/1 -> Mux2/2
  after2/1 -> Demux2/1
  Demux2/3 -> Rate Transition6/1  "P_batt_driver [w]"
  Demux2/1 -> Rate Transition4/1  "P-eng [W]"
  Demux2/2 -> Rate Transition5/1  "eng-mode-"
  Gain/1 -> Mux2/4
  Horizon_Lowlayer [s]/1 -> Mux2/1
  Mux2/1 -> Rate Transition1/1
  SOC [%]/1 -> Gain/1
  Interpreted MATLAB Function2/1 -> after2/1
  Rate Transition1/1 -> Interpreted MATLAB Function2/1
  Rate Transition5/1 -> engine speed/2(Engine Mode 2-Work 1-No Work)  "eng-mode-"
  Rate Transition4/1 -> engine speed/1(Engine Power Demand (W))  "P-eng [W]"
  Rate Transition6/1 -> motor control1/5, engine speed/3(Pch)  "P_batt_driver [w]"

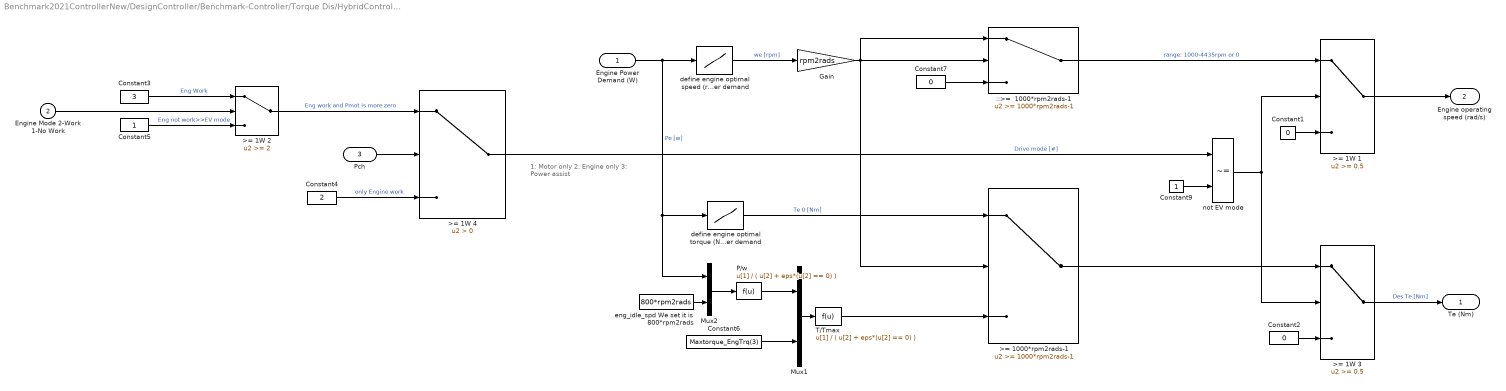
== system Benchmark2021ControllerNew/DesignController/Benchmark-Controller/Torque Dis/HybridController/Drive/PMP-based S-function/engine speed ==
  note: 1: Motor only
      | 2: Engine only
      | 3: Power assist
  Engine Power Demand (W) : Inport
  Engine Mode 2-Work 1-No Work : Inport  Port=2
  Pch : Inport  Port=3
  ::>=  1000*rpm2rads-1 : Switch  Threshold=1000*rpm2rads-1  SaturateOnIntegerOverflow=on  InputSameDT=on
  >= 1000*rpm2rads-1 : Switch  Threshold=1000*rpm2rads-1  SaturateOnIntegerOverflow=on  InputSameDT=on
  >= 1W 1 : Switch  Threshold=0.5  SaturateOnIntegerOverflow=on  InputSameDT=on
  >= 1W 2 : Switch  Threshold=2  SaturateOnIntegerOverflow=on  InputSameDT=on
  >= 1W 3 : Switch  Threshold=0.5  SaturateOnIntegerOverflow=on  InputSameDT=on
  >= 1W 4 : Switch  Criteria=u2 > Threshold  SaturateOnIntegerOverflow=on  InputSameDT=on
  Constant1 : Constant  Value=0
  Constant2 : Constant  Value=0
  Constant3 : Constant  Value=3
  Constant4 : Constant  Value=2
  Constant5 : Constant
  Constant6 : Constant  Value=Maxtorque_EngTrq(3)
  Constant7 : Constant  Value=0
  Constant9 : Constant
  Gain : Gain  Gain=rpm2rads
  Mux1 : Mux  Inputs=2
  Mux2 : Mux  Inputs=2
  P/w : Fcn  Expr=u[1] / ( u[2] + eps*(u[2] == 0) )
  T/Tmax : Fcn  Expr=u[1] / ( u[2] + eps*(u[2] == 0) )
  define engine optimal speed (rpm) base on power demand : Lookup  InputValues=Power_level  Table=N_opt  SaturateOnIntegerOverflow=on
  define engine optimal torque (Nm) base on power demand : Lookup  InputValues=Power_level  Table=T_opt  SaturateOnIntegerOverflow=on
  eng_idle_spd We set it is 800*rpm2rads : Constant  Value=800*rpm2rads
  not EV mode : RelationalOperator  Operator=~=  RndMeth=Nearest  InputSameDT=on
  Te (Nm) : Outport
  Engine operating speed (rad/s) : Outport  Port=2
  wires:
  define engine optimal speed (rpm) base on power demand/1 -> Gain/1  "we [rpm]"
  Engine Power Demand (W)/1 -> define engine optimal speed (rpm) base on power demand/1, define engine optimal torque (Nm) base on power demand/1, Mux2/1  "Pe [w]"
  >= 1W 3/1 -> Te (Nm)/1  "Des Te [Nm]"
  define engine optimal torque (Nm) base on power demand/1 -> >= 1000*rpm2rads-1/1  "Te 0 [Nm]"
  Constant1/1 -> >= 1W 1/3
  >= 1W 1/1 -> Engine operating speed (rad/s)/1
  >= 1000*rpm2rads-1/1 -> >= 1W 3/1
  Gain/1 -> >= 1000*rpm2rads-1/2, ::>=  1000*rpm2rads-1/2, ::>=  1000*rpm2rads-1/1
  T/Tmax/1 -> >= 1000*rpm2rads-1/3
  ::>=  1000*rpm2rads-1/1 -> >= 1W 1/1  "range: 1000-4435rpm or 0"
  Constant2/1 -> >= 1W 3/3
  not EV mode/1 -> >= 1W 1/2, >= 1W 3/2
  Constant9/1 -> not EV mode/2
  >= 1W 4/1 -> not EV mode/1  "Drive mode [#]"
  Mux2/1 -> P/w/1
  Mux1/1 -> T/Tmax/1
  Constant6/1 -> Mux1/2
  eng_idle_spd We set it is 800*rpm2rads/1 -> Mux2/2
  P/w/1 -> Mux1/1
  Constant7/1 -> ::>=  1000*rpm2rads-1/3
  Constant4/1 -> >= 1W 4/3  "only Engine work"
  >= 1W 2/1 -> >= 1W 4/1  "Eng work and Pmot is more zero"
  Pch/1 -> >= 1W 4/2
  Engine Mode 2-Work 1-No Work/1 -> >= 1W 2/2
  Constant5/1 -> >= 1W 2/3  "Eng not work>>EV mode"
  Constant3/1 -> >= 1W 2/1  "Eng Work"

== system Benchmark2021ControllerNew/DesignController/Benchmark-Controller/Torque Dis/HybridController/Drive/PMP-based S-function/tire2mg2 ==
  Spd_Veh_Des_km/h : Inport
  Km/h>>m/s : Gain  Gain=1/3.6
  "Rt : mm" : Gain  Gain=1/Rt*1000
  tx_pg_r/tx_pg_s1 : Gain  Gain=Rf2/Rf1  SaturateOnIntegerOverflow=on  OutDataTypeStr=Inherit: Same as input  ParamDataTypeStr=Inherit: Same as input
  tx_pg_r/tx_pg_s2 : Gain  Gain=Rc2/Rm  SaturateOnIntegerOverflow=on  OutDataTypeStr=Inherit: Same as input  ParamDataTypeStr=Inherit: Same as input
  Omg_mg2_Des_rads : Outport
  wires:
  "Rt : mm"/1 -> tx_pg_r/tx_pg_s1/1
  Km/h>>m/s/1 -> "Rt : mm"/1
  Spd_Veh_Des_km/h/1 -> Km/h>>m/s/1
  tx_pg_r/tx_pg_s2/1 -> Omg_mg2_Des_rads/1
  tx_pg_r/tx_pg_s1/1 -> tx_pg_r/tx_pg_s2/1

== matlab function Benchmark2021ControllerNew/DesignController/Benchmark-Controller/Speed Planning/MATLAB Function3 ==
  data: u input; y output
function y = fcn(u)

y = u(3:end-1,1);

== matlab function Benchmark2021ControllerNew/DesignController/Benchmark-Controller/Torque Dis/Driver Model/Power_cal/Cal_des_TQ_Omega_P(now) ==
  settings: updateMethod=DISCRETE  sampleTime=0.05
  data: N_des_req_now output; M_des_req_now output; v_des_req_seq input; slope_des_req_seq input; P_des_req_now output; Horizon_Lowlayer parameter; Sampling_Lowlayer parameter; N_PMP_Lowlayer parameter
function [N_des_req_now,M_des_req_now,P_des_req_now] = fcn(v_des_req_seq,slope_des_req_seq,Horizon_Lowlayer, Sampling_Lowlayer, N_PMP_Lowlayer)
%% Parameter of Prediction
% Horizon = 2;%Prediction Horizon 0.05-4 [s]
Horizon= Horizon_Lowlayer;% Prediction Horizon 0.05-4 [s]
Sampling = Sampling_Lowlayer;%0.1 [s]
N_PMP = N_PMP_Lowlayer;
%% Input
v_des_req_kmph = v_des_req_seq;%unit [km/h]
slope_des_req_rad = slope_des_req_seq;%it is a direct output [rad]
%% parameters
v_des_req=zeros(N_PMP,1);% unit:[m/s]
v_des_req(1:end)=v_des_req_kmph(1:end)*1000/3600;% We use the unit [m/s]
% Vehicle parameters
Rf2=75;Rf1=19;
epsilon=Rf2/Rf1;% reduction ratio [-]
Rw=317.25/1000;%radius [m]
beltaCA=0.0291*3.6*3.6;% because beltaCA*v_req(i-1)^2 in it v_req:[km/h] -> so:we use [m/s]
Mveh=1700;% the mass of vehicle [kg]
Mvehg=9.807;%g
mu=0.006434;% Coefficient of roll [-]
eta4=0.97;% efficiency [-]
%% slope
Slope_des_dist_now=slope_des_req_rad(1);
%% desired Omega now (for Driver PID)
v_req_seq_now=v_des_req(1);% now v_des unit:[m/s]
v_req_seq_next=v_des_req(2);% next time v_des unit:[m/s]
sigma_des_now=Slope_des_dist_now;% now slope unit:[rad]
Nreq_des_now=v_req_seq_now*epsilon*60/(2*pi*Rw);%rpm,,because 1rad/s = 60*1/(2*3.1415) rpm = 9.55 rpm
Nreq2Power_now=Nreq_des_now/9549;%it help to get power[kw] easily. Because [rpm*Nm/9550=kw]
%% desired Torque & Power now (for Driver PID)
a_req0=(v_req_seq_next-v_req_seq_now)/Sampling;%m/s^2
Ffric_a0=a_req0*Mveh;
Ffric_mu0=mu*Mveh*Mvehg*cos(sigma_des_now);
Ffric_s0 =Mveh*Mvehg*sin(sigma_des_now);
Ffric_v0=beltaCA*v_req_seq_now^2;
Ffric0=Ffric_a0 + Ffric_mu0 + Ffric_s0 + Ffric_v0;%行驶阻力
Mreq_des_now=Ffric0*Rw/epsilon/eta4;%Nm
P_des_now=Nreq2Power_now*Mreq_des_now;
%% stop state
% if v_req_seq_now==0
%     if Ffric_s0>Ffric_mu0
%         P_des_now=abs(Ffric_s0)-abs(Ffric_mu0);
%     else
%         P_des_now=0;
%     end
% end
%% Output
P_des_req_now=P_des_now;
N_des_req_now=Nreq_des_now;
M_des_req_now=Mreq_des_now;

== matlab function Benchmark2021ControllerNew/DesignController/Benchmark-Controller/Speed Planning/SignalNum Calcu ==
  data: ego_distance input size=1; N_inter_h output size=1; N_inter_pre output size=1; preceding_distance input
function [N_inter_h,N_inter_pre] = fcn(ego_distance,preceding_distance)

intersection = [1288;
2358;
2572;
2886;
3066;
3150;
3422;
3784;
4696;
5377;
5576;
6855;
7626;
10162;
10575;
10948;
11201;
11537;
11781;
12302;
12587;
12785;
13032;
13368;
14364;
15802]; % original position of the intersection to the departure


intersection = intersection-3.2; 
% the vehicle length should be considered at the departure 
% and at the departure, the distance of ego vehicle to the first intesection is actually 1284.8 [m]
% so a correction of 3.2 [m] is given.

if ego_distance < intersection(1)
    N_inter_h = 1;
elseif ego_distance < intersection(2)
    N_inter_h = 2;
elseif ego_distance < intersection(3)
    N_inter_h = 3;
elseif ego_distance < intersection(4)
    N_inter_h = 4;
elseif ego_distance < intersection(5)
    N_inter_h = 5;
elseif ego_distance < intersection(6)
    N_inter_h = 6;
elseif ego_distance < intersection(7)
    N_inter_h = 7;
elseif ego_distance < intersection(8)
    N_inter_h = 8;
elseif ego_distance < intersection(9)
    N_inter_h = 9;
elseif ego_distance < intersection(10)
    N_inter_h = 10;
elseif ego_distance < intersection(11)
    N_inter_h = 11;
elseif ego_distance < intersection(12)
    N_inter_h = 12;
elseif ego_distance < intersection(13)
    N_inter_h = 13;
elseif ego_distance < intersection(14)
    N_inter_h = 14;
elseif ego_distance < intersection(15)
    N_inter_h = 15;
elseif ego_distance < intersection(16)
    N_inter_h = 16;
elseif ego_distance < intersection(17)
    N_inter_h = 17;
elseif ego_distance < intersection(18)
    N_inter_h = 18;
elseif ego_distance < intersection(19)
    N_inter_h = 19;
elseif ego_distance < intersection(20)
    N_inter_h = 20;
elseif ego_distance < intersection(21)
    N_inter_h = 21;
elseif ego_distance < intersection(22)
    N_inter_h = 22;
elseif ego_distance < intersection(23)
    N_inter_h = 23;
elseif ego_distance < intersection(24)
    N_inter_h = 24;
elseif ego_distance < intersection(25)
    N_inter_h = 25;
elseif ego_distance < intersection(26)
    N_inter_h = 26;
else
    N_inter_h = 27;
end

if preceding_distance < intersection(1)
    N_inter_pre = 1;
elseif preceding_distance < intersection(2)
    N_inter_pre = 2;
elseif preceding_distance < intersection(3)
    N_inter_pre = 3;
elseif preceding_distance < intersection(4)
    N_inter_pre = 4;
elseif preceding_distance < intersection(5)
    N_inter_pre = 5;
elseif preceding_distance < intersection(6)
    N_inter_pre = 6;
elseif preceding_distance < intersection(7)
    N_inter_pre = 7;
elseif preceding_distance < intersection(8)
    N_inter_pre = 8;
elseif preceding_distance < intersection(9)
    N_inter_pre = 9;
elseif preceding_distance < intersection(10)
    N_inter_pre = 10;
elseif preceding_distance < intersection(11)
    N_inter_pre = 11;
elseif preceding_distance < intersection(12)
    N_inter_pre = 12;
elseif preceding_distance < intersection(13)
    N_inter_pre = 13;
elseif preceding_distance < intersection(14)
    N_inter_pre = 14;
elseif preceding_distance < intersection(15)
    N_inter_pre = 15;
elseif preceding_distance < intersection(16)
    N_inter_pre = 16;
elseif preceding_distance < intersection(17)
    N_inter_pre = 17;
elseif preceding_distance < intersection(18)
    N_inter_pre = 18;
elseif preceding_distance < intersection(19)
    N_inter_pre = 19;
elseif preceding_distance < intersection(20)
    N_inter_pre = 20;
elseif preceding_distance < intersection(21)
    N_inter_pre = 21;
elseif preceding_distance < intersection(22)
    N_inter_pre = 22;
elseif preceding_distance < intersection(23)
    N_inter_pre = 23;
elseif preceding_distance < intersection(24)
    N_inter_pre = 24;
elseif preceding_distance < intersection(25)
    N_inter_pre = 25;
elseif preceding_distance < intersection(26)
    N_inter_pre = 26;
else
    N_inter_pre = 27;
end

== matlab function Benchmark2021ControllerNew/DesignController/Benchmark-Controller/Torque Dis/Driver Model/Power_cal/Power_Seq ==
  data: Input_Horizon input size=1; Output_P_seq output; Input_Sampling input; Input_vh_seq input; Input_P_PID input; Input_N_des_now input; Input_TQ_des_now input; Input_Slope_seq input
function Output_P_seq = fcn(Input_Horizon,Input_Sampling,Input_vh_seq,Input_P_PID,Input_N_des_now,Input_TQ_des_now,Input_Slope_seq)
%% Parameter of Prediction
%% Input
Horizon = Input_Horizon;%Prediction Horizon 0.05-4 [s]
Sampling = Input_Sampling;% Prediction Horizon 0.05-4 [s]
N_PMP = Horizon/Sampling;
% N_PMP = single(Horizon/Sampling);
% v_des_req_kmph = Input_vh_seq;%unit [km/h]
v_des_req = Input_vh_seq;%unit [m/s]
Preq_real_pidout_now = Input_P_PID;%it is a direct output [kw]
Nreq_des_now = Input_N_des_now;
Mreq_des_now = Input_TQ_des_now;
Slope_des_dist = Input_Slope_seq;
%% parameters
% v_des_req=zeros(N_PMP,1);% unit:[m/s]
% v_des_req(1:end)=v_des_req_kmph(1:end)*1000/3600;% We use the unit [m/s]
% Vehicle parameters
Rf2=75;Rf1=19;
epsilon=Rf2/Rf1;% reduction ratio [-]
Rw=317.25/1000;%radius [m]
beltaCA=0.0291*3.6*3.6;% because beltaCA*v_req(i-1)^2 in it v_req:[km/h] -> so:we use [m/s]
Mveh=1700;% the mass of vehicle [kg]
Mvehg=9.807;%g
mu=0.006434;% Coefficient of roll [-]
eta4=0.97;% efficiency [-]
%% Predict future Power (for MPC)
% Preq = zeros(N_PMP,1);% unit:[kw]
% Mreq = zeros(N_PMP,1);% unit:[Nm]
% Nreq = zeros(N_PMP,1);% unit:[rpm]
Preq = zeros(70,1);% unit:[kw]%%%%%%%%%%%%%%%%%%%%%%%%%%%%%%%%%%%%%
Mreq = zeros(70,1);% unit:[Nm]%%%%%%%%%%%%%%%%%%%%%%%%%%%%%%%%%%%%%%%%%%%%
Nreq = zeros(70,1);% unit:[rpm]%%%%%%%%%%%%%%%%%%%%%%%%%%%%%%%%%%%%%%%%%%%%%%%
Mreq(1)=Mreq_des_now;
Nreq(1)=Nreq_des_now;
Preq(1) = Preq_real_pidout_now;% unit:[kw]
for i = 2:1:N_PMP   %
    sigma= Slope_des_dist(i-1);
    a_req=(v_des_req(i)-v_des_req(i-1))/Sampling;%m/s2
    Ffric_a=a_req*Mveh;
    Ffric_mu=mu*Mveh*Mvehg*cos(sigma);
    Ffric_s=Mveh*Mvehg*sin(sigma);
    Ffric_v=beltaCA*v_des_req(i-1)^2;
    Ffric=Ffric_a + Ffric_mu + Ffric_s + Ffric_v;%all of the 
    Mreq(i)=Ffric*Rw/epsilon/eta4;%Nm
    Nreq(i)=v_des_req(i)*epsilon*60/(2*pi*Rw);% [rpm] Because:1 rad/s=60/(2*pi) rpm = 9.55 rpm
    Preq(i) =Mreq(i).*Nreq(i)/9549;%kw
end
%% Output
% Power_req_seq=Preq(1:N_PMP,1);
% y=[Power_req_seq];
% Output_P_seq=Preq(1:N_PMP,1);
Output_P_seq=Preq;
